simulink model "flightControlSystem"  (R2021a)
settings: Solver=ode3  StartTime=0  StopTime=TFinal  FixedStep=Ts  RelTol=1e-3  EnableMultiTasking=on
undefined symbols (not defined in the file): codertarget, Controller, DiscIntNeverNeededParam, Discrete, Estimator, g, gray, init, Sensors, Time, Ts, var_acc_angle_N, var_bias_gyr_N, var_gyro_p_N, Vehicle
libraries: simulink x39, pid_lib x4, ctrlSharedLib x4, sharedtransform x3, parrotlib x1
(part 4 of 4)

== matlab function flightControlSystem/Control System/Controller/Position Controller/Position error transformation (Earth to Body frame) ==
  data: yaw input; xy_err_earth input; xy_err_body output
function xy_err_body = fcn(yaw,xy_err_earth)

transformation = [cos(yaw), sin(yaw); -sin(yaw),  cos(yaw)];
xy_err_body = transformation * xy_err_earth;


end

== stateflow chart flightControlSystem/Control System/Path Planning/Chart ==
  state MoveStraight
    during:
    xout=xout+0.000010*x_new;
    yout=yout+0.000010*y_new;
    zout=zout;
  state Circle_detected
    during:
    xout=xout+0.000035*x_new;
    yout=yout+0.000035*y_new;
    zout=zout;
  state Land
    during:
    xout=xout;
    yout=yout;
    zout=zout+0.01;
  state Hover
    entry:
    xout=xestim;
    yout=yestim;
    zout=-1.1;
  state MoveStraight1
    during:
    xout=xout+0.000005*x_new ;
    yout=yout+0.000005*y_new ;
    zout=zout;
  state Land1
    during:
    xout=xout;
    yout=yout;
    zout=0;
  Hover -> MoveStraight : [after(3,sec)]
  MoveStraight -> Circle_detected [order 2] : [circle_detect == 1]
  Circle_detected -> Land : [circle_detect == 0]
  (default) -> Hover
  Land -> Land1 : [zout >= -0.1]
  MoveStraight -> MoveStraight1 [order 1] : [corner_detected == 1]
  MoveStraight1 -> MoveStraight [order 1] : [corner_detected == 0]
  MoveStraight1 -> Circle_detected [order 2] : [circle_detect == 1]
  data: xestim input; yestim input; y_new input; xout output single; yout output single; zout output single; x_new input; corner_detected input; circle_detect input
